simulink model "model"  (R2022a)
settings: Solver=FixedStepAuto  StartTime=0.0  StopTime=5  FixedStep=0.001  RelTol=1e-3
PreLoadFcn:
  | A1 = 4;
  | f1 = pi;
  | A2 = 3;
  | f2 = pi/2;
settings Model: Creator=DNE  LastModifiedBy=DNE

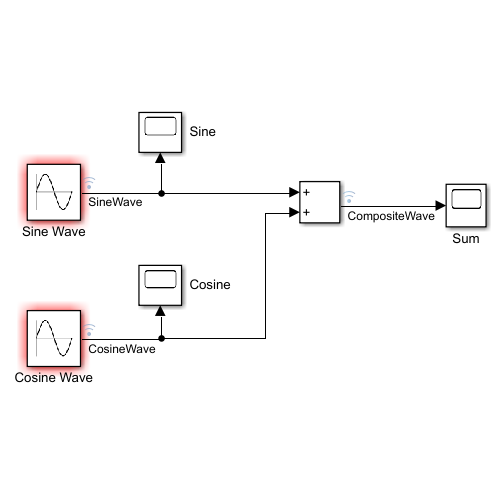
[thumbnail: Simulink's stored preview of the top-level diagram]
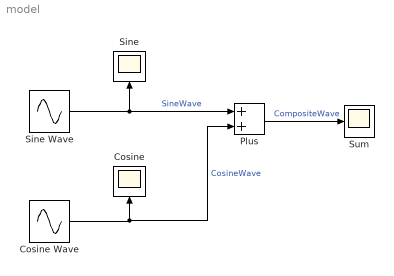
== system model ==
  Cosine : Scope
  Cosine Wave : Sin  Amplitude=A2  Frequency=f2  Phase=pi/2  SampleTime=0
  Plus : Sum
  Sine : Scope
  Sine Wave : Sin  Amplitude=A1  Frequency=f1  SampleTime=0
  Sum : Scope
  wires:
  Sine Wave/1 -> Plus/1, Sine/1  "SineWave"
  Cosine Wave/1 -> Plus/2, Cosine/1  "CosineWave"
  Plus/1 -> Sum/1  "CompositeWave"
